simulink model "diff_drive_robot_pid_system"  (R2025a)
settings: Solver=ode45  StartTime=0.0  StopTime=20  RelTol=1e-3
undefined symbols (not defined in the file or in its folder): ROBOT_DIST_FORCE_GAIN, ROBOT_DIST_TORQUE_GAIN, ROBOT_EPS, ROBOT_FORCE_GAIN, ROBOT_LEFT_LOAD_BIAS, ROBOT_MOTOR_GAIN, ROBOT_MOTOR_TAU, ROBOT_RIGHT_LOAD_BIAS, ROBOT_SENSOR_THRESHOLD, ROBOT_TARGET_X, ROBOT_TARGET_Y, ROBOT_THETA_KD, ROBOT_THETA_KI, ROBOT_THETA_KP, ROBOT_WHEEL_BASE, ROBOT_WHEEL_KD, ROBOT_WHEEL_KI, ROBOT_WHEEL_KP, ROBOT_WHEEL_RADIUS, ROBOT_XY_GAIN
libraries: slpidlib x3, simulink x1
settings Model: Creator=wzy  LastModifiedBy=wzy

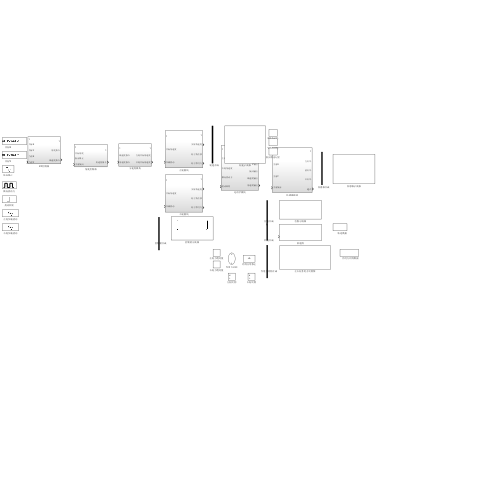
[thumbnail: Simulink's stored preview of the top-level diagram]
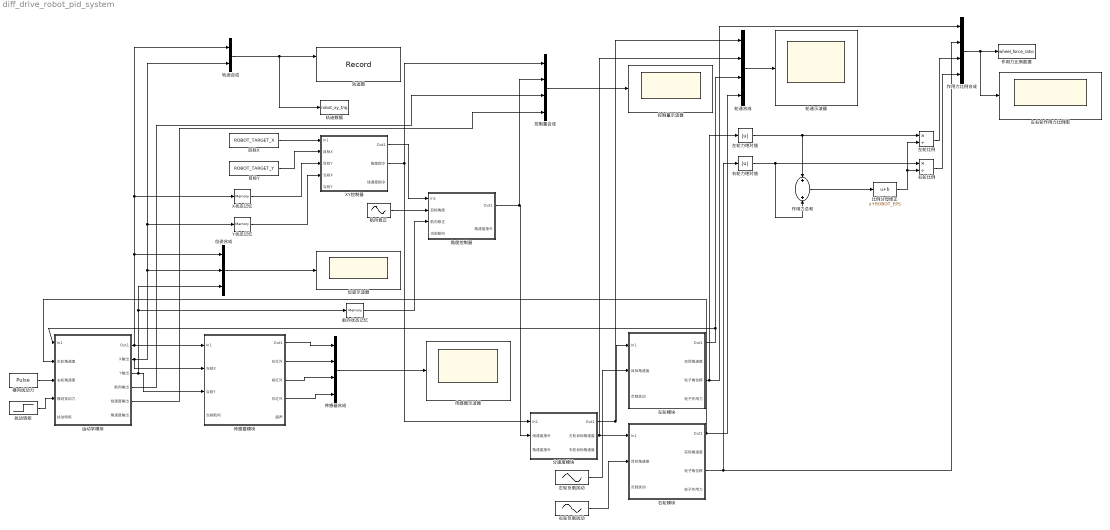
== system diff_drive_robot_pid_system ==
  XY控制器 : Subsystem
      settings: AttributesFormatString=输出: 角度指令, 线速度指令
  X状态记忆 : Memory
  Y状态记忆 : Memory
  传感器合成 : Mux
  传感器模块 : Subsystem
      settings: AttributesFormatString=输出: 左红外, 前红外, 右红外, 超声
  传感器示波器 : Scope
  位姿合成 : Mux  Inputs=3
  位姿示波器 : Scope
  作用力总和 : Sum
  作用力比例合成 : Mux
  作用力比例数据 : ToWorkspace  VariableName=wheel_force_ratio  SaveFormat=Structure With Time  SampleTime=-1
  分速度模块 : Subsystem
      settings: AttributesFormatString=输出: 左右轮目标角速度
  右轮力绝对值 : Abs  SaturateOnIntegerOverflow=off
  右轮模块 : Subsystem
      settings: AttributesFormatString=输入: 目标角速度, 负载扰动; 输出: 角速度, 角位移, 作用力
  右轮比例 : Product  Inputs=*/
  右轮负载扰动 : Sin  Amplitude=0.22  Bias=ROBOT_RIGHT_LOAD_BIAS  Frequency=0.82  SampleTime=0
  左右轮作用力比例图 : Scope
  左轮力绝对值 : Abs  SaturateOnIntegerOverflow=off
  左轮模块 : Subsystem
      settings: AttributesFormatString=输入: 目标角速度, 负载扰动; 输出: 角速度, 角位移, 作用力
  左轮比例 : Product  Inputs=*/
  左轮负载扰动 : Sin  Amplitude=0.28  Bias=ROBOT_LEFT_LOAD_BIAS  Frequency=1.15  SampleTime=0
  扰动转矩 : Step  Time=6  After=0.6  SampleTime=0
  控制量合成 : Mux
  控制量示波器 : Scope
  横向扰动力 : DiscretePulseGenerator  PulseType=Time based  Amplitude=2  Period=20  PulseWidth=15
  比例分母修正 : Bias  Bias=ROBOT_EPS  SaturateOnIntegerOverflow=off
  目标X : Constant  Value=ROBOT_TARGET_X
  目标Y : Constant  Value=ROBOT_TARGET_Y
  航向修正 : Sin  Amplitude=0.45  Frequency=0.55  SampleTime=0
  航向状态记忆 : Memory
  角度控制器 : Subsystem
      settings: AttributesFormatString=输出: 角速度指令
  轨迹合成 : Mux  Inputs=2
  轨迹图 : Record  NumPorts=2.0  FileSettingsInternal="{\"entries\":[{\"content\":{\"excelSettings\":{\"content\":{},\"type\":\"Streamout.ExcelSettings\"},\"parquetSettings\":{\"content\":{},\"type\":\"Streamout.ParquetSettings\"}},\"type\":\"Streamout.FileSettingStorage\",\"uuid\":\"\"}],\"packageUris\":[\"http:\\/\\/schema.mathworks.com\\/mf0\\/streamout_blocks\\/R2020a\"],\"version\":\"1.0\"}"  FrameSettings=[0, 0]  Layout=[1 1]  SignalsInternal="{\"entries\":[{\"content\":{\"signals\":[{\"content\":{\"blockPath\":[],\"dimensions\":[1],\"domain\":\"\",\"lineColor\":\"#a2142f\",\"plots\":[ 1 ],\"port\":1,\"signalID\":1,\"signalName\":\"XY Graph:1\"},\"type\":\"RecordBlkView.Signal\",\"uuid\":\"\"},{\"content\":{\"blockPath\":[],\"dimensions\":[1],\"domain\":\"\",\"lineColor\":\"#139fff\",\"plots\":[ 1 ],\"port\":2,\"signalID\":2,\"signalName\":\"XY Graph:2\"},\"type\":\"RecordBlkView.Signal\",\"uuid\":\"\"}]},\"type\":\"RecordBlkView.InputSignals\",\"uuid\":\"\"}],\"packageUris\":[\"http:\\/\\/schema.mathworks.com\\/mf0\\/streamout_blocks\\/R2020a\"],\"version\":\"1.0\"}"  VisualizationBindings="{\"xyplotplugin\":{\"info\":[{\"series\":[{\"bindingParametersList\":[{\"parameter\":\"X-Axis\",\"signalID\":1,\"signalName\":\"XY Graph:1\"},{\"parameter\":\"Y-Axis\",\"signalID\":2,\"signalName\":\"XY Graph:2\"}],\"seriesID\":0}],\"subplotID\":1}]}}"  CompatibilityTag=XY
  轨迹数据 : ToWorkspace  VariableName=robot_xy_traj  SaveFormat=Structure With Time  SampleTime=-1
  轮速合成 : Mux
  轮速示波器 : Scope
  运动学模块 : Subsystem
      settings: AttributesFormatString=输入: 左轮, 右轮, 外力, 转矩; 输出: X, Y, 航向, v, w
  wires:
  传感器合成/1 -> 传感器示波器/1
  运动学模块/5(线速度输出) -> 控制量合成/4
  右轮模块/3(轮子角位移) -> 作用力比例合成/2, 右轮力绝对值/1
  横向扰动力/1 -> 运动学模块/3(右轮角速度)
  目标X/1 -> XY控制器/1(In1)
  轨迹合成/1 -> 轨迹图/1, 轨迹数据/1
  扰动转矩/1 -> 运动学模块/4(横向扰动力)
  分速度模块/1(Out1) -> 轮速合成/1, 左轮模块/1(In1)
  运动学模块/1(Out1) -> X状态记忆/1, 轨迹合成/1, 位姿合成/1, 传感器模块/1(In1)
  运动学模块/2(X输出) -> Y状态记忆/1, 轨迹合成/2, 位姿合成/2, 传感器模块/2(当前X)
  作用力总和/1 -> 比例分母修正/1
  运动学模块/3(Y输出) -> 航向状态记忆/1, 位姿合成/3, 传感器模块/3(当前Y)
  运动学模块/4(航向输出) -> 控制量合成/3
  目标Y/1 -> XY控制器/2(目标X)
  X状态记忆/1 -> XY控制器/3(目标Y)
  右轮比例/1 -> 作用力比例合成/4
  左轮负载扰动/1 -> 左轮模块/2(目标角速度)
  Y状态记忆/1 -> XY控制器/4(当前X)
  位姿合成/1 -> 位姿示波器/1
  传感器模块/1(Out1) -> 传感器合成/1
  航向修正/1 -> 角度控制器/2(目标角度)
  传感器模块/2(左红外) -> 传感器合成/2
  传感器模块/3(前红外) -> 传感器合成/3
  传感器模块/4(右红外) -> 传感器合成/4
  比例分母修正/1 -> 左轮比例/2, 右轮比例/2
  XY控制器/1(Out1) -> 角度控制器/1(In1)
  XY控制器/2(角度指令) -> 分速度模块/1(In1), 控制量合成/1
  航向状态记忆/1 -> 角度控制器/3(航向修正)
  角度控制器/1(Out1) -> 分速度模块/2(线速度指令), 控制量合成/2
  控制量合成/1 -> 控制量示波器/1
  分速度模块/2(左轮目标角速度) -> 轮速合成/2, 右轮模块/1(In1)
  作用力比例合成/1 -> 左右轮作用力比例图/1, 作用力比例数据/1
  右轮负载扰动/1 -> 右轮模块/2(目标角速度)
  左轮模块/1(Out1) -> 轮速合成/3, 运动学模块/1(In1)
  左轮模块/3(轮子角位移) -> 作用力比例合成/1, 左轮力绝对值/1
  右轮模块/1(Out1) -> 轮速合成/4, 运动学模块/2(左轮角速度)
  轮速合成/1 -> 轮速示波器/1
  左轮力绝对值/1 -> 作用力总和/1, 左轮比例/1
  右轮力绝对值/1 -> 作用力总和/2, 右轮比例/1
  左轮比例/1 -> 作用力比例合成/3

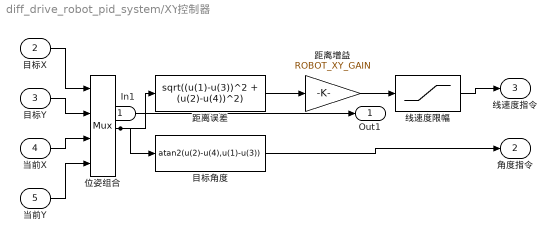
== system diff_drive_robot_pid_system/XY控制器 ==
  In1 : Inport
  目标X : Inport  Port=2
  目标Y : Inport  Port=3
  当前X : Inport  Port=4
  当前Y : Inport  Port=5
  位姿组合 : Mux
  目标角度 : Fcn  Expr=atan2(u(2)-u(4),u(1)-u(3))
  线速度限幅 : Saturate  UpperLimit=0.8  LowerLimit=-0.8
  距离增益 : Gain  Gain=ROBOT_XY_GAIN
  距离误差 : Fcn  Expr=sqrt((u(1)-u(3))^2 + (u(2)-u(4))^2)
  Out1 : Outport
  角度指令 : Outport  Port=2
  线速度指令 : Outport  Port=3
  wires:
  In1/1 -> Out1/1
  目标X/1 -> 位姿组合/1
  目标Y/1 -> 位姿组合/2
  当前X/1 -> 位姿组合/3
  当前Y/1 -> 位姿组合/4
  位姿组合/1 -> 距离误差/1, 目标角度/1
  距离误差/1 -> 距离增益/1
  距离增益/1 -> 线速度限幅/1
  线速度限幅/1 -> 线速度指令/1
  目标角度/1 -> 角度指令/1

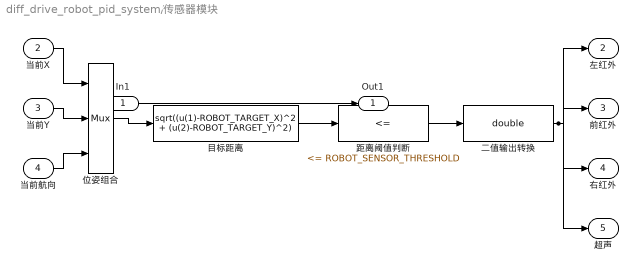
== system diff_drive_robot_pid_system/传感器模块 ==
  In1 : Inport
  当前X : Inport  Port=2
  当前Y : Inport  Port=3
  当前航向 : Inport  Port=4
  二值输出转换 : DataTypeConversion  OutDataTypeStr=double  SaturateOnIntegerOverflow=off  RndMeth=Floor
  位姿组合 : Mux  Inputs=3
  目标距离 : Fcn  Expr=sqrt((u(1)-ROBOT_TARGET_X)^2 + (u(2)-ROBOT_TARGET_Y)^2)
  距离阈值判断 : simulink/Logic and Bit Operations/Compare To Constant  relop=<=  const=ROBOT_SENSOR_THRESHOLD  OutDataTypeStr=boolean
  Out1 : Outport
  左红外 : Outport  Port=2
  前红外 : Outport  Port=3
  右红外 : Outport  Port=4
  超声 : Outport  Port=5
  wires:
  In1/1 -> Out1/1
  当前X/1 -> 位姿组合/1
  当前Y/1 -> 位姿组合/2
  当前航向/1 -> 位姿组合/3
  位姿组合/1 -> 目标距离/1
  目标距离/1 -> 距离阈值判断/1
  距离阈值判断/1 -> 二值输出转换/1
  二值输出转换/1 -> 左红外/1, 前红外/1, 右红外/1, 超声/1

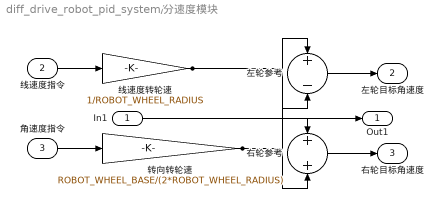
== system diff_drive_robot_pid_system/分速度模块 ==
  In1 : Inport
  线速度指令 : Inport  Port=2
  角速度指令 : Inport  Port=3
  右轮参考 : Sum
  左轮参考 : Sum  Inputs=+-
  线速度转轮速 : Gain  Gain=1/ROBOT_WHEEL_RADIUS
  转向转轮速 : Gain  Gain=ROBOT_WHEEL_BASE/(2*ROBOT_WHEEL_RADIUS)
  Out1 : Outport
  左轮目标角速度 : Outport  Port=2
  右轮目标角速度 : Outport  Port=3
  wires:
  In1/1 -> Out1/1
  线速度指令/1 -> 线速度转轮速/1
  角速度指令/1 -> 转向转轮速/1
  线速度转轮速/1 -> 左轮参考/1, 右轮参考/1
  转向转轮速/1 -> 左轮参考/2, 右轮参考/2
  左轮参考/1 -> 左轮目标角速度/1
  右轮参考/1 -> 右轮目标角速度/1

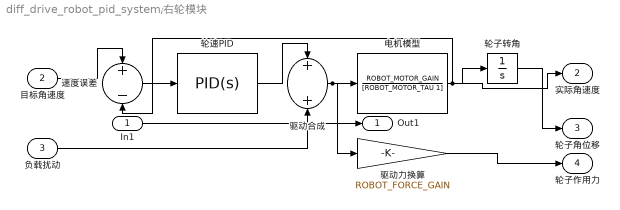
== system diff_drive_robot_pid_system/右轮模块 ==
  In1 : Inport
  目标角速度 : Inport  Port=2
  负载扰动 : Inport  Port=3
  电机模型 : TransferFcn  Numerator=ROBOT_MOTOR_GAIN  Denominator=[ROBOT_MOTOR_TAU 1]
  轮子转角 : Integrator
  轮速PID : slpidlib/PID Controller  Controller=PID  Form=Parallel  TimeDomain=Continuous-time  UseExternalTs=off  SampleTime=-1  IntegratorMethod=Forward Euler  FilterMethod=Forward Euler  ControllerParametersSource=internal  P=ROBOT_WHEEL_KP  I=ROBOT_WHEEL_KI  UseKiTs=off  D=ROBOT_WHEEL_KD  UseExternalDerivativeSource=off  N=100  UseFilter=on  TunerSelectOption=Transfer Function Based (PID Tuner App)  InitialConditionSource=internal  InitialConditionForIntegrator=0  InitialConditionForFilter=0  DifferentiatorICPrevScaledInput=0  ExternalReset=none  TrackingMode=off  Kt=1  LimitOutput=off  SatLimitsSource=internal  UpperSaturationLimit=inf  LowerSaturationLimit=-inf  LinearizeAsGain=on  AntiWindupMode=none  Kb=1  LimitIntegrator=off  UpperIntegratorSaturationLimit=inf  LowerIntegratorSaturationLimit=-inf  POutMin=[]  POutMax=[]  IOutMin=[]  IOutMax=[]  DOutMin=[]  DOutMax=[]  NOutMin=[]  NOutMax=[]  SumOutMin=[]  SumOutMax=[]  SaturationOutMin=[]  SaturationOutMax=[]  PParamMin=[]  PParamMax=[]  IParamMin=[]  IParamMax=[]  DParamMin=[]  DParamMax=[]  NParamMin=[]  NParamMax=[]  KbParamMin=[]  KbParamMax=[]  KtParamMin=[]  KtParamMax=[]  KbOutMin=[]  KbOutMax=[]  KtOutMin=[]  KtOutMax=[]  IntegratorOutMin=[]  IntegratorOutMax=[]  FilterOutMin=[]  FilterOutMax=[]  SumI1OutMin=[]  SumI1OutMax=[]  SumI2OutMin=[]  SumI2OutMax=[]  SumI3OutMin=[]  SumI3OutMax=[]  SumI4OutMin=[]  SumI4OutMax=[]  SumDOutMin=[]  SumDOutMax=[]  DifferentiatorOutMin=[]  DifferentiatorOutMax=[]  FilterDiffOutCoefMin=[]  FilterDiffOutCoefMax=[]  ReciprocalOutMin=[]  ReciprocalOutMax=[]  SumDenOutMin=[]  SumDenOutMax=[]  SumNumOutMin=[]  SumNumOutMax=[]  DivideOutMin=[]  DivideOutMax=[]  UdiffTsProdOutMin=[]  UdiffTsProdOutMax=[]  NTsProdOutMin=[]  NTsProdOutMax=[]  UintegralTsProdOutMin=[]  UintegralTsProdOutMax=[]  UngainTsProdOutMin=[]  UngainTsProdOutMax=[]  ClampingZeroOutDataTypeStr=Inherit: Inherit via back propagation  ClampingZeroOutMin=[]  ClampingZeroOutMax=[]  FilterDenConstantOutDataTypeStr=Inherit: Inherit via back propagation  FilterDenConstantOutMin=[]  FilterDenConstantOutMax=[]  PCopyOutDataTypeStr=Inherit: Inherit via back propagation  PCopyOutMin=[]  PCopyOutMax=[]  NCopyOutDataTypeStr=Inherit: Inherit via back propagation  NCopyOutMin=[]  NCopyOutMax=[]  IntegratorContinuousStateAttributes=''  IntegratorStateMustResolveToSignalObject=off  IntegratorRTWStateStorageClass=Auto  FilterContinuousStateAttributes=''  FilterStateMustResolveToSignalObject=off  FilterRTWStateStorageClass=Auto  ParallelPVariant=InternalParameters  IdealPVariant=Disabled  IVariant=InternalParameters  DVariant=InternalParameters  IntegratorVariant=Continuous  SatVariant=Disabled  AWVariant=Passthrough  PCopyVariant=Disabled  TRVariant=Disabled  FdbkBlocksVariant=Forward  IdealPFdbkVariant=Disabled  SatFdbkVariant=Disabled  DerivativeFilterVariant=ContFilter  NVariant=InternalParameters  NCopyVariant=Disabled  FilterICVariant=InternalICsFilter  IntegratorICVariant=InternalICs  ExternalResetVariant=Disabled  TRSumVariant=Passthrough  SumFdbkVariant=Disabled  SumVariant=Sum_PID  TsampFilterVariant=InternalTs  TsampNgainVariant=Passthrough  TsampIntegralVariant=Disabled_SignalSpec  ExternalSaturationOutDataTypeStr=Inherit: Same as second input  DerivativeSourceVariant=ErrorSignal  PreIntVariant=InternalPreInt
  速度误差 : Sum  Inputs=+-
  驱动力换算 : Gain  Gain=ROBOT_FORCE_GAIN
  驱动合成 : Sum
  Out1 : Outport
  实际角速度 : Outport  Port=2
  轮子角位移 : Outport  Port=3
  轮子作用力 : Outport  Port=4
  wires:
  In1/1 -> Out1/1
  目标角速度/1 -> 速度误差/1
  速度误差/1 -> 轮速PID/1
  轮速PID/1 -> 驱动合成/1
  负载扰动/1 -> 驱动合成/2
  驱动合成/1 -> 电机模型/1, 驱动力换算/1
  电机模型/1 -> 速度误差/2, 轮子转角/1, 实际角速度/1
  轮子转角/1 -> 轮子角位移/1
  驱动力换算/1 -> 轮子作用力/1

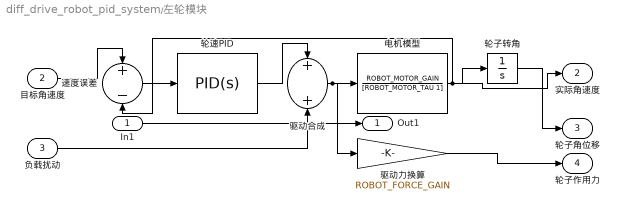
== system diff_drive_robot_pid_system/左轮模块 ==
  In1 : Inport
  目标角速度 : Inport  Port=2
  负载扰动 : Inport  Port=3
  电机模型 : TransferFcn  Numerator=ROBOT_MOTOR_GAIN  Denominator=[ROBOT_MOTOR_TAU 1]
  轮子转角 : Integrator
  轮速PID : slpidlib/PID Controller  Controller=PID  Form=Parallel  TimeDomain=Continuous-time  UseExternalTs=off  SampleTime=-1  IntegratorMethod=Forward Euler  FilterMethod=Forward Euler  ControllerParametersSource=internal  P=ROBOT_WHEEL_KP  I=ROBOT_WHEEL_KI  UseKiTs=off  D=ROBOT_WHEEL_KD  UseExternalDerivativeSource=off  N=100  UseFilter=on  TunerSelectOption=Transfer Function Based (PID Tuner App)  InitialConditionSource=internal  InitialConditionForIntegrator=0  InitialConditionForFilter=0  DifferentiatorICPrevScaledInput=0  ExternalReset=none  TrackingMode=off  Kt=1  LimitOutput=off  SatLimitsSource=internal  UpperSaturationLimit=inf  LowerSaturationLimit=-inf  LinearizeAsGain=on  AntiWindupMode=none  Kb=1  LimitIntegrator=off  UpperIntegratorSaturationLimit=inf  LowerIntegratorSaturationLimit=-inf  POutMin=[]  POutMax=[]  IOutMin=[]  IOutMax=[]  DOutMin=[]  DOutMax=[]  NOutMin=[]  NOutMax=[]  SumOutMin=[]  SumOutMax=[]  SaturationOutMin=[]  SaturationOutMax=[]  PParamMin=[]  PParamMax=[]  IParamMin=[]  IParamMax=[]  DParamMin=[]  DParamMax=[]  NParamMin=[]  NParamMax=[]  KbParamMin=[]  KbParamMax=[]  KtParamMin=[]  KtParamMax=[]  KbOutMin=[]  KbOutMax=[]  KtOutMin=[]  KtOutMax=[]  IntegratorOutMin=[]  IntegratorOutMax=[]  FilterOutMin=[]  FilterOutMax=[]  SumI1OutMin=[]  SumI1OutMax=[]  SumI2OutMin=[]  SumI2OutMax=[]  SumI3OutMin=[]  SumI3OutMax=[]  SumI4OutMin=[]  SumI4OutMax=[]  SumDOutMin=[]  SumDOutMax=[]  DifferentiatorOutMin=[]  DifferentiatorOutMax=[]  FilterDiffOutCoefMin=[]  FilterDiffOutCoefMax=[]  ReciprocalOutMin=[]  ReciprocalOutMax=[]  SumDenOutMin=[]  SumDenOutMax=[]  SumNumOutMin=[]  SumNumOutMax=[]  DivideOutMin=[]  DivideOutMax=[]  UdiffTsProdOutMin=[]  UdiffTsProdOutMax=[]  NTsProdOutMin=[]  NTsProdOutMax=[]  UintegralTsProdOutMin=[]  UintegralTsProdOutMax=[]  UngainTsProdOutMin=[]  UngainTsProdOutMax=[]  ClampingZeroOutDataTypeStr=Inherit: Inherit via back propagation  ClampingZeroOutMin=[]  ClampingZeroOutMax=[]  FilterDenConstantOutDataTypeStr=Inherit: Inherit via back propagation  FilterDenConstantOutMin=[]  FilterDenConstantOutMax=[]  PCopyOutDataTypeStr=Inherit: Inherit via back propagation  PCopyOutMin=[]  PCopyOutMax=[]  NCopyOutDataTypeStr=Inherit: Inherit via back propagation  NCopyOutMin=[]  NCopyOutMax=[]  IntegratorContinuousStateAttributes=''  IntegratorStateMustResolveToSignalObject=off  IntegratorRTWStateStorageClass=Auto  FilterContinuousStateAttributes=''  FilterStateMustResolveToSignalObject=off  FilterRTWStateStorageClass=Auto  ParallelPVariant=InternalParameters  IdealPVariant=Disabled  IVariant=InternalParameters  DVariant=InternalParameters  IntegratorVariant=Continuous  SatVariant=Disabled  AWVariant=Passthrough  PCopyVariant=Disabled  TRVariant=Disabled  FdbkBlocksVariant=Forward  IdealPFdbkVariant=Disabled  SatFdbkVariant=Disabled  DerivativeFilterVariant=ContFilter  NVariant=InternalParameters  NCopyVariant=Disabled  FilterICVariant=InternalICsFilter  IntegratorICVariant=InternalICs  ExternalResetVariant=Disabled  TRSumVariant=Passthrough  SumFdbkVariant=Disabled  SumVariant=Sum_PID  TsampFilterVariant=InternalTs  TsampNgainVariant=Passthrough  TsampIntegralVariant=Disabled_SignalSpec  ExternalSaturationOutDataTypeStr=Inherit: Same as second input  DerivativeSourceVariant=ErrorSignal  PreIntVariant=InternalPreInt
  速度误差 : Sum  Inputs=+-
  驱动力换算 : Gain  Gain=ROBOT_FORCE_GAIN
  驱动合成 : Sum
  Out1 : Outport
  实际角速度 : Outport  Port=2
  轮子角位移 : Outport  Port=3
  轮子作用力 : Outport  Port=4
  wires:
  In1/1 -> Out1/1
  目标角速度/1 -> 速度误差/1
  速度误差/1 -> 轮速PID/1
  轮速PID/1 -> 驱动合成/1
  负载扰动/1 -> 驱动合成/2
  驱动合成/1 -> 电机模型/1, 驱动力换算/1
  电机模型/1 -> 速度误差/2, 轮子转角/1, 实际角速度/1
  轮子转角/1 -> 轮子角位移/1
  驱动力换算/1 -> 轮子作用力/1

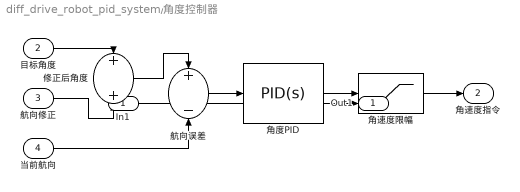
== system diff_drive_robot_pid_system/角度控制器 ==
  In1 : Inport
  目标角度 : Inport  Port=2
  航向修正 : Inport  Port=3
  当前航向 : Inport  Port=4
  修正后角度 : Sum
  航向误差 : Sum  Inputs=+-
  角度PID : slpidlib/PID Controller  Controller=PID  Form=Parallel  TimeDomain=Continuous-time  UseExternalTs=off  SampleTime=-1  IntegratorMethod=Forward Euler  FilterMethod=Forward Euler  ControllerParametersSource=internal  P=ROBOT_THETA_KP  I=ROBOT_THETA_KI  UseKiTs=off  D=ROBOT_THETA_KD  UseExternalDerivativeSource=off  N=100  UseFilter=on  TunerSelectOption=Transfer Function Based (PID Tuner App)  InitialConditionSource=internal  InitialConditionForIntegrator=0  InitialConditionForFilter=0  DifferentiatorICPrevScaledInput=0  ExternalReset=none  TrackingMode=off  Kt=1  LimitOutput=off  SatLimitsSource=internal  UpperSaturationLimit=inf  LowerSaturationLimit=-inf  LinearizeAsGain=on  AntiWindupMode=none  Kb=1  LimitIntegrator=off  UpperIntegratorSaturationLimit=inf  LowerIntegratorSaturationLimit=-inf  POutMin=[]  POutMax=[]  IOutMin=[]  IOutMax=[]  DOutMin=[]  DOutMax=[]  NOutMin=[]  NOutMax=[]  SumOutMin=[]  SumOutMax=[]  SaturationOutMin=[]  SaturationOutMax=[]  PParamMin=[]  PParamMax=[]  IParamMin=[]  IParamMax=[]  DParamMin=[]  DParamMax=[]  NParamMin=[]  NParamMax=[]  KbParamMin=[]  KbParamMax=[]  KtParamMin=[]  KtParamMax=[]  KbOutMin=[]  KbOutMax=[]  KtOutMin=[]  KtOutMax=[]  IntegratorOutMin=[]  IntegratorOutMax=[]  FilterOutMin=[]  FilterOutMax=[]  SumI1OutMin=[]  SumI1OutMax=[]  SumI2OutMin=[]  SumI2OutMax=[]  SumI3OutMin=[]  SumI3OutMax=[]  SumI4OutMin=[]  SumI4OutMax=[]  SumDOutMin=[]  SumDOutMax=[]  DifferentiatorOutMin=[]  DifferentiatorOutMax=[]  FilterDiffOutCoefMin=[]  FilterDiffOutCoefMax=[]  ReciprocalOutMin=[]  ReciprocalOutMax=[]  SumDenOutMin=[]  SumDenOutMax=[]  SumNumOutMin=[]  SumNumOutMax=[]  DivideOutMin=[]  DivideOutMax=[]  UdiffTsProdOutMin=[]  UdiffTsProdOutMax=[]  NTsProdOutMin=[]  NTsProdOutMax=[]  UintegralTsProdOutMin=[]  UintegralTsProdOutMax=[]  UngainTsProdOutMin=[]  UngainTsProdOutMax=[]  ClampingZeroOutDataTypeStr=Inherit: Inherit via back propagation  ClampingZeroOutMin=[]  ClampingZeroOutMax=[]  FilterDenConstantOutDataTypeStr=Inherit: Inherit via back propagation  FilterDenConstantOutMin=[]  FilterDenConstantOutMax=[]  PCopyOutDataTypeStr=Inherit: Inherit via back propagation  PCopyOutMin=[]  PCopyOutMax=[]  NCopyOutDataTypeStr=Inherit: Inherit via back propagation  NCopyOutMin=[]  NCopyOutMax=[]  IntegratorContinuousStateAttributes=''  IntegratorStateMustResolveToSignalObject=off  IntegratorRTWStateStorageClass=Auto  FilterContinuousStateAttributes=''  FilterStateMustResolveToSignalObject=off  FilterRTWStateStorageClass=Auto  ParallelPVariant=InternalParameters  IdealPVariant=Disabled  IVariant=InternalParameters  DVariant=InternalParameters  IntegratorVariant=Continuous  SatVariant=Disabled  AWVariant=Passthrough  PCopyVariant=Disabled  TRVariant=Disabled  FdbkBlocksVariant=Forward  IdealPFdbkVariant=Disabled  SatFdbkVariant=Disabled  DerivativeFilterVariant=ContFilter  NVariant=InternalParameters  NCopyVariant=Disabled  FilterICVariant=InternalICsFilter  IntegratorICVariant=InternalICs  ExternalResetVariant=Disabled  TRSumVariant=Passthrough  SumFdbkVariant=Disabled  SumVariant=Sum_PID  TsampFilterVariant=InternalTs  TsampNgainVariant=Passthrough  TsampIntegralVariant=Disabled_SignalSpec  ExternalSaturationOutDataTypeStr=Inherit: Same as second input  DerivativeSourceVariant=ErrorSignal  PreIntVariant=InternalPreInt
  角速度限幅 : Saturate  UpperLimit=1.5  LowerLimit=-1.5
  Out1 : Outport
  角速度指令 : Outport  Port=2
  wires:
  In1/1 -> Out1/1
  目标角度/1 -> 修正后角度/1
  航向修正/1 -> 修正后角度/2
  修正后角度/1 -> 航向误差/1
  当前航向/1 -> 航向误差/2
  航向误差/1 -> 角度PID/1
  角度PID/1 -> 角速度限幅/1
  角速度限幅/1 -> 角速度指令/1

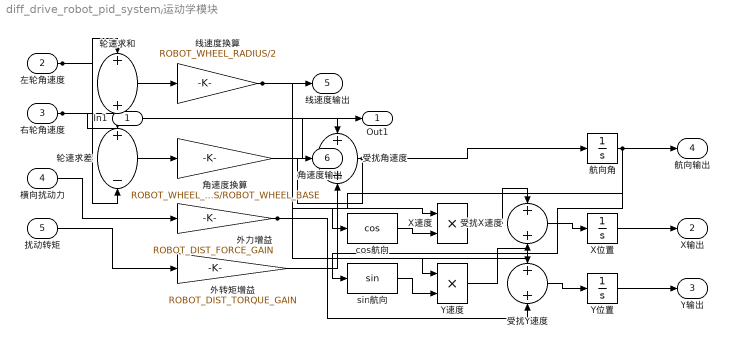
== system diff_drive_robot_pid_system/运动学模块 ==
  In1 : Inport
  左轮角速度 : Inport  Port=2
  右轮角速度 : Inport  Port=3
  横向扰动力 : Inport  Port=4
  扰动转矩 : Inport  Port=5
  X位置 : Integrator
  X速度 : Product  Inputs=**
  Y位置 : Integrator
  Y速度 : Product  Inputs=**
  cos航向 : Trigonometry  Operator=cos
  sin航向 : Trigonometry
  受扰X速度 : Sum
  受扰Y速度 : Sum
  受扰角速度 : Sum
  外力增益 : Gain  Gain=ROBOT_DIST_FORCE_GAIN
  外转矩增益 : Gain  Gain=ROBOT_DIST_TORQUE_GAIN
  线速度换算 : Gain  Gain=ROBOT_WHEEL_RADIUS/2
  航向角 : Integrator
  角速度换算 : Gain  Gain=ROBOT_WHEEL_RADIUS/ROBOT_WHEEL_BASE
  轮速求和 : Sum
  轮速求差 : Sum  Inputs=+-
  Out1 : Outport
  X输出 : Outport  Port=2
  Y输出 : Outport  Port=3
  航向输出 : Outport  Port=4
  线速度输出 : Outport  Port=5
  角速度输出 : Outport  Port=6
  wires:
  In1/1 -> Out1/1
  左轮角速度/1 -> 轮速求和/1, 轮速求差/2
  右轮角速度/1 -> 轮速求和/2, 轮速求差/1
  轮速求和/1 -> 线速度换算/1
  轮速求差/1 -> 角速度换算/1
  横向扰动力/1 -> 外力增益/1
  扰动转矩/1 -> 外转矩增益/1
  角速度换算/1 -> 受扰角速度/1
  外转矩增益/1 -> 受扰角速度/2
  线速度换算/1 -> 线速度输出/1, X速度/1, Y速度/1
  受扰角速度/1 -> 角速度输出/1, 航向角/1
  航向角/1 -> 航向输出/1, cos航向/1, sin航向/1
  cos航向/1 -> X速度/2
  sin航向/1 -> Y速度/2
  X速度/1 -> 受扰X速度/1
  外力增益/1 -> 受扰X速度/2, 受扰Y速度/2
  Y速度/1 -> 受扰Y速度/1
  受扰X速度/1 -> X位置/1
  X位置/1 -> X输出/1
  受扰Y速度/1 -> Y位置/1
  Y位置/1 -> Y输出/1
